simulink model "NUgus_IK"  (R2018a)
settings: Solver=VariableStepAuto  StartTime=0.0  StopTime=inf  RelTol=1e-3
values from neighbouring files (symbols this model uses):
  CM740_acc_bias = 4 * 9.80743    (= 39.22972)    [CM740_init.m]
  CM740_acc_gain = 512 / CM740_acc_centre    [CM740_init.m]
  CM740_gyro_bias = 1600 / 360 * 2 * pi    (= 27.9252680319)    [CM740_init.m]
  CM740_gyro_gain = 512 / CM740_gyro_centre    [CM740_init.m]
  head = [-0.05482228998067195, -0.00010888238321339966, 0.0011712900228573724, 0.41900000000000004]    [comtest.m]
  s = mean(abs(present_speed.data))    [RunServoTest.m]
  torso = [0.0050079703254699804, 0.008880921777563762, 0.1021503146237477, 2.5390000000000006]    [comtest.m]
undefined symbols (not defined in the file or in its folder): floor, X, Y, Z
libraries: sm_lib x211, fl_lib x128, nesl_utility x68
(part 8 of 8)

== system NUgus_IK/NUgus/left_foot/foot_fl_contact/calculate forces/x contact force ==
  PS Max1 : fl_lib/Physical Signals/Nonlinear Operators/PS Max
      settings: SourceProductName=Simscape  SourceProductBaseCode=SS
  PS Min1 : fl_lib/Physical Signals/Nonlinear Operators/PS Min
      settings: SourceProductName=Simscape  SourceProductBaseCode=SS
  PS Switch : fl_lib/Physical Signals/Nonlinear Operators/PS Switch  Threshold=0
      settings: SourceProductName=Simscape  SourceProductBaseCode=SS
  frictionless : PMIOPort  Side=Left
  force : PMIOPort  Port=2  Side=Right
  velocity : PMIOPort  Port=3  Side=Left
  z position : PMIOPort  Port=4  Side=Left
  upper_bound : PMIOPort  Port=5  Side=Left
  lower_bound : PMIOPort  Port=6  Side=Left
  connections:
  PS Max1/LConn2 -- lower_bound/RConn1
  PS Max1/LConn1 -- PS Min1/RConn1
  PS Switch/LConn3 -- PS Max1/RConn1
  PS Min1/LConn1 -- velocity/RConn1
  PS Switch/LConn2 -- z position/RConn1
  PS Switch/LConn1 -- frictionless/RConn1
  PS Switch/RConn1 -- force/RConn1
  upper_bound/RConn1 -- PS Min1/LConn2

== system NUgus_IK/NUgus/left_foot/foot_fl_contact/calculate forces/y contact force ==
  PS Max1 : fl_lib/Physical Signals/Nonlinear Operators/PS Max
      settings: SourceProductName=Simscape  SourceProductBaseCode=SS
  PS Min1 : fl_lib/Physical Signals/Nonlinear Operators/PS Min
      settings: SourceProductName=Simscape  SourceProductBaseCode=SS
  PS Switch : fl_lib/Physical Signals/Nonlinear Operators/PS Switch  Threshold=0
      settings: SourceProductName=Simscape  SourceProductBaseCode=SS
  frictionless : PMIOPort  Side=Left
  force : PMIOPort  Port=2  Side=Right
  velocity : PMIOPort  Port=3  Side=Left
  z position : PMIOPort  Port=4  Side=Left
  upper_bound : PMIOPort  Port=5  Side=Left
  lower_bound : PMIOPort  Port=6  Side=Left
  connections:
  PS Max1/LConn2 -- lower_bound/RConn1
  PS Max1/LConn1 -- PS Min1/RConn1
  PS Switch/LConn3 -- PS Max1/RConn1
  PS Min1/LConn1 -- velocity/RConn1
  PS Switch/LConn2 -- z position/RConn1
  PS Switch/LConn1 -- frictionless/RConn1
  PS Switch/RConn1 -- force/RConn1
  upper_bound/RConn1 -- PS Min1/LConn2

== system NUgus_IK/NUgus/left_foot/foot_fr_contact/calculate forces/x contact force ==
  PS Max1 : fl_lib/Physical Signals/Nonlinear Operators/PS Max
      settings: SourceProductName=Simscape  SourceProductBaseCode=SS
  PS Min1 : fl_lib/Physical Signals/Nonlinear Operators/PS Min
      settings: SourceProductName=Simscape  SourceProductBaseCode=SS
  PS Switch : fl_lib/Physical Signals/Nonlinear Operators/PS Switch  Threshold=0
      settings: SourceProductName=Simscape  SourceProductBaseCode=SS
  frictionless : PMIOPort  Side=Left
  force : PMIOPort  Port=2  Side=Right
  velocity : PMIOPort  Port=3  Side=Left
  z position : PMIOPort  Port=4  Side=Left
  upper_bound : PMIOPort  Port=5  Side=Left
  lower_bound : PMIOPort  Port=6  Side=Left
  connections:
  PS Max1/LConn2 -- lower_bound/RConn1
  PS Max1/LConn1 -- PS Min1/RConn1
  PS Switch/LConn3 -- PS Max1/RConn1
  PS Min1/LConn1 -- velocity/RConn1
  PS Switch/LConn2 -- z position/RConn1
  PS Switch/LConn1 -- frictionless/RConn1
  PS Switch/RConn1 -- force/RConn1
  upper_bound/RConn1 -- PS Min1/LConn2

== system NUgus_IK/NUgus/left_foot/foot_fr_contact/calculate forces/y contact force ==
  PS Max1 : fl_lib/Physical Signals/Nonlinear Operators/PS Max
      settings: SourceProductName=Simscape  SourceProductBaseCode=SS
  PS Min1 : fl_lib/Physical Signals/Nonlinear Operators/PS Min
      settings: SourceProductName=Simscape  SourceProductBaseCode=SS
  PS Switch : fl_lib/Physical Signals/Nonlinear Operators/PS Switch  Threshold=0
      settings: SourceProductName=Simscape  SourceProductBaseCode=SS
  frictionless : PMIOPort  Side=Left
  force : PMIOPort  Port=2  Side=Right
  velocity : PMIOPort  Port=3  Side=Left
  z position : PMIOPort  Port=4  Side=Left
  upper_bound : PMIOPort  Port=5  Side=Left
  lower_bound : PMIOPort  Port=6  Side=Left
  connections:
  PS Max1/LConn2 -- lower_bound/RConn1
  PS Max1/LConn1 -- PS Min1/RConn1
  PS Switch/LConn3 -- PS Max1/RConn1
  PS Min1/LConn1 -- velocity/RConn1
  PS Switch/LConn2 -- z position/RConn1
  PS Switch/LConn1 -- frictionless/RConn1
  PS Switch/RConn1 -- force/RConn1
  upper_bound/RConn1 -- PS Min1/LConn2

== system NUgus_IK/NUgus/right_foot/foot_bl_contact/calculate forces/x contact force ==
  PS Max1 : fl_lib/Physical Signals/Nonlinear Operators/PS Max
      settings: SourceProductName=Simscape  SourceProductBaseCode=SS
  PS Min1 : fl_lib/Physical Signals/Nonlinear Operators/PS Min
      settings: SourceProductName=Simscape  SourceProductBaseCode=SS
  PS Switch : fl_lib/Physical Signals/Nonlinear Operators/PS Switch  Threshold=0
      settings: SourceProductName=Simscape  SourceProductBaseCode=SS
  frictionless : PMIOPort  Side=Left
  force : PMIOPort  Port=2  Side=Right
  velocity : PMIOPort  Port=3  Side=Left
  z position : PMIOPort  Port=4  Side=Left
  upper_bound : PMIOPort  Port=5  Side=Left
  lower_bound : PMIOPort  Port=6  Side=Left
  connections:
  PS Max1/LConn2 -- lower_bound/RConn1
  PS Max1/LConn1 -- PS Min1/RConn1
  PS Switch/LConn3 -- PS Max1/RConn1
  PS Min1/LConn1 -- velocity/RConn1
  PS Switch/LConn2 -- z position/RConn1
  PS Switch/LConn1 -- frictionless/RConn1
  PS Switch/RConn1 -- force/RConn1
  upper_bound/RConn1 -- PS Min1/LConn2

== system NUgus_IK/NUgus/right_foot/foot_bl_contact/calculate forces/y contact force ==
  PS Max1 : fl_lib/Physical Signals/Nonlinear Operators/PS Max
      settings: SourceProductName=Simscape  SourceProductBaseCode=SS
  PS Min1 : fl_lib/Physical Signals/Nonlinear Operators/PS Min
      settings: SourceProductName=Simscape  SourceProductBaseCode=SS
  PS Switch : fl_lib/Physical Signals/Nonlinear Operators/PS Switch  Threshold=0
      settings: SourceProductName=Simscape  SourceProductBaseCode=SS
  frictionless : PMIOPort  Side=Left
  force : PMIOPort  Port=2  Side=Right
  velocity : PMIOPort  Port=3  Side=Left
  z position : PMIOPort  Port=4  Side=Left
  upper_bound : PMIOPort  Port=5  Side=Left
  lower_bound : PMIOPort  Port=6  Side=Left
  connections:
  PS Max1/LConn2 -- lower_bound/RConn1
  PS Max1/LConn1 -- PS Min1/RConn1
  PS Switch/LConn3 -- PS Max1/RConn1
  PS Min1/LConn1 -- velocity/RConn1
  PS Switch/LConn2 -- z position/RConn1
  PS Switch/LConn1 -- frictionless/RConn1
  PS Switch/RConn1 -- force/RConn1
  upper_bound/RConn1 -- PS Min1/LConn2

== system NUgus_IK/NUgus/right_foot/foot_br_contact/calculate forces/x contact force ==
  PS Max1 : fl_lib/Physical Signals/Nonlinear Operators/PS Max
      settings: SourceProductName=Simscape  SourceProductBaseCode=SS
  PS Min1 : fl_lib/Physical Signals/Nonlinear Operators/PS Min
      settings: SourceProductName=Simscape  SourceProductBaseCode=SS
  PS Switch : fl_lib/Physical Signals/Nonlinear Operators/PS Switch  Threshold=0
      settings: SourceProductName=Simscape  SourceProductBaseCode=SS
  frictionless : PMIOPort  Side=Left
  force : PMIOPort  Port=2  Side=Right
  velocity : PMIOPort  Port=3  Side=Left
  z position : PMIOPort  Port=4  Side=Left
  upper_bound : PMIOPort  Port=5  Side=Left
  lower_bound : PMIOPort  Port=6  Side=Left
  connections:
  PS Max1/LConn2 -- lower_bound/RConn1
  PS Max1/LConn1 -- PS Min1/RConn1
  PS Switch/LConn3 -- PS Max1/RConn1
  PS Min1/LConn1 -- velocity/RConn1
  PS Switch/LConn2 -- z position/RConn1
  PS Switch/LConn1 -- frictionless/RConn1
  PS Switch/RConn1 -- force/RConn1
  upper_bound/RConn1 -- PS Min1/LConn2

== system NUgus_IK/NUgus/right_foot/foot_br_contact/calculate forces/y contact force ==
  PS Max1 : fl_lib/Physical Signals/Nonlinear Operators/PS Max
      settings: SourceProductName=Simscape  SourceProductBaseCode=SS
  PS Min1 : fl_lib/Physical Signals/Nonlinear Operators/PS Min
      settings: SourceProductName=Simscape  SourceProductBaseCode=SS
  PS Switch : fl_lib/Physical Signals/Nonlinear Operators/PS Switch  Threshold=0
      settings: SourceProductName=Simscape  SourceProductBaseCode=SS
  frictionless : PMIOPort  Side=Left
  force : PMIOPort  Port=2  Side=Right
  velocity : PMIOPort  Port=3  Side=Left
  z position : PMIOPort  Port=4  Side=Left
  upper_bound : PMIOPort  Port=5  Side=Left
  lower_bound : PMIOPort  Port=6  Side=Left
  connections:
  PS Max1/LConn2 -- lower_bound/RConn1
  PS Max1/LConn1 -- PS Min1/RConn1
  PS Switch/LConn3 -- PS Max1/RConn1
  PS Min1/LConn1 -- velocity/RConn1
  PS Switch/LConn2 -- z position/RConn1
  PS Switch/LConn1 -- frictionless/RConn1
  PS Switch/RConn1 -- force/RConn1
  upper_bound/RConn1 -- PS Min1/LConn2

== system NUgus_IK/NUgus/right_foot/foot_fl_contact/calculate forces/x contact force ==
  PS Max1 : fl_lib/Physical Signals/Nonlinear Operators/PS Max
      settings: SourceProductName=Simscape  SourceProductBaseCode=SS
  PS Min1 : fl_lib/Physical Signals/Nonlinear Operators/PS Min
      settings: SourceProductName=Simscape  SourceProductBaseCode=SS
  PS Switch : fl_lib/Physical Signals/Nonlinear Operators/PS Switch  Threshold=0
      settings: SourceProductName=Simscape  SourceProductBaseCode=SS
  frictionless : PMIOPort  Side=Left
  force : PMIOPort  Port=2  Side=Right
  velocity : PMIOPort  Port=3  Side=Left
  z position : PMIOPort  Port=4  Side=Left
  upper_bound : PMIOPort  Port=5  Side=Left
  lower_bound : PMIOPort  Port=6  Side=Left
  connections:
  PS Max1/LConn2 -- lower_bound/RConn1
  PS Max1/LConn1 -- PS Min1/RConn1
  PS Switch/LConn3 -- PS Max1/RConn1
  PS Min1/LConn1 -- velocity/RConn1
  PS Switch/LConn2 -- z position/RConn1
  PS Switch/LConn1 -- frictionless/RConn1
  PS Switch/RConn1 -- force/RConn1
  upper_bound/RConn1 -- PS Min1/LConn2

== system NUgus_IK/NUgus/right_foot/foot_fl_contact/calculate forces/y contact force ==
  PS Max1 : fl_lib/Physical Signals/Nonlinear Operators/PS Max
      settings: SourceProductName=Simscape  SourceProductBaseCode=SS
  PS Min1 : fl_lib/Physical Signals/Nonlinear Operators/PS Min
      settings: SourceProductName=Simscape  SourceProductBaseCode=SS
  PS Switch : fl_lib/Physical Signals/Nonlinear Operators/PS Switch  Threshold=0
      settings: SourceProductName=Simscape  SourceProductBaseCode=SS
  frictionless : PMIOPort  Side=Left
  force : PMIOPort  Port=2  Side=Right
  velocity : PMIOPort  Port=3  Side=Left
  z position : PMIOPort  Port=4  Side=Left
  upper_bound : PMIOPort  Port=5  Side=Left
  lower_bound : PMIOPort  Port=6  Side=Left
  connections:
  PS Max1/LConn2 -- lower_bound/RConn1
  PS Max1/LConn1 -- PS Min1/RConn1
  PS Switch/LConn3 -- PS Max1/RConn1
  PS Min1/LConn1 -- velocity/RConn1
  PS Switch/LConn2 -- z position/RConn1
  PS Switch/LConn1 -- frictionless/RConn1
  PS Switch/RConn1 -- force/RConn1
  upper_bound/RConn1 -- PS Min1/LConn2

== system NUgus_IK/NUgus/right_foot/foot_fr_contact/calculate forces/x contact force ==
  PS Max1 : fl_lib/Physical Signals/Nonlinear Operators/PS Max
      settings: SourceProductName=Simscape  SourceProductBaseCode=SS
  PS Min1 : fl_lib/Physical Signals/Nonlinear Operators/PS Min
      settings: SourceProductName=Simscape  SourceProductBaseCode=SS
  PS Switch : fl_lib/Physical Signals/Nonlinear Operators/PS Switch  Threshold=0
      settings: SourceProductName=Simscape  SourceProductBaseCode=SS
  frictionless : PMIOPort  Side=Left
  force : PMIOPort  Port=2  Side=Right
  velocity : PMIOPort  Port=3  Side=Left
  z position : PMIOPort  Port=4  Side=Left
  upper_bound : PMIOPort  Port=5  Side=Left
  lower_bound : PMIOPort  Port=6  Side=Left
  connections:
  PS Max1/LConn2 -- lower_bound/RConn1
  PS Max1/LConn1 -- PS Min1/RConn1
  PS Switch/LConn3 -- PS Max1/RConn1
  PS Min1/LConn1 -- velocity/RConn1
  PS Switch/LConn2 -- z position/RConn1
  PS Switch/LConn1 -- frictionless/RConn1
  PS Switch/RConn1 -- force/RConn1
  upper_bound/RConn1 -- PS Min1/LConn2

== system NUgus_IK/NUgus/right_foot/foot_fr_contact/calculate forces/y contact force ==
  PS Max1 : fl_lib/Physical Signals/Nonlinear Operators/PS Max
      settings: SourceProductName=Simscape  SourceProductBaseCode=SS
  PS Min1 : fl_lib/Physical Signals/Nonlinear Operators/PS Min
      settings: SourceProductName=Simscape  SourceProductBaseCode=SS
  PS Switch : fl_lib/Physical Signals/Nonlinear Operators/PS Switch  Threshold=0
      settings: SourceProductName=Simscape  SourceProductBaseCode=SS
  frictionless : PMIOPort  Side=Left
  force : PMIOPort  Port=2  Side=Right
  velocity : PMIOPort  Port=3  Side=Left
  z position : PMIOPort  Port=4  Side=Left
  upper_bound : PMIOPort  Port=5  Side=Left
  lower_bound : PMIOPort  Port=6  Side=Left
  connections:
  PS Max1/LConn2 -- lower_bound/RConn1
  PS Max1/LConn1 -- PS Min1/RConn1
  PS Switch/LConn3 -- PS Max1/RConn1
  PS Min1/LConn1 -- velocity/RConn1
  PS Switch/LConn2 -- z position/RConn1
  PS Switch/LConn1 -- frictionless/RConn1
  PS Switch/RConn1 -- force/RConn1
  upper_bound/RConn1 -- PS Min1/LConn2

== matlab function NUgus_IK/Forward Kinematics/Simulink Function/FK Function ==
  data: HtRSp output; p input; HtLSp output; HtRSr output; HtLSr output; HtRE output; HtLE output; HtRHy output; HtLHy output; HtRHr output; HtLHr output; HtRHp output; HtLHp output; HtRK output; HtLK output; HtRAp output; HtLAp output; HtRAr output; HtLAr output; HtHy output; HtHp output
function [HtRSp, HtLSp, HtRSr, HtLSr, HtRE, HtLE, HtRHy, HtLHy, HtRHr, HtLHr, HtRHp, HtLHp, HtRK, HtLK, HtRAp, HtLAp, HtRAr, HtLAr, HtHy, HtHp] = FK(p)
    model = NUgusKinematics();

    kinematics = Kinematics(model);
    
    % Get FK for arms
    [RSp, RSr, RE] = kinematics.armFK(p, false);
    [LSp, LSr, LE] = kinematics.armFK(p, true);
    % Get FK for legs
    [RHy, RHr, RHp, RK, RAp, RAr] = kinematics.legFK(p, false);
    [LHy, LHr, LHp, LK, LAp, LAr] = kinematics.legFK(p, true);
    % Get FK for Head
    [Hy, Hp] = kinematics.headFK(p);
    
    % Return FK in servo order
    HtRSp = RSp.tf;
    HtLSp = LSp.tf;
    HtRSr = RSr.tf;
    HtLSr = LSr.tf;
    HtRE = RE.tf;
    HtLE = LE.tf;
    HtRHy = RHy.tf;
    HtLHy = LHy.tf;
    HtRHr = RHr.tf;
    HtLHr = LHr.tf;
    HtRHp = RHp.tf;
    HtLHp = LHp.tf;
    HtRK = RK.tf;
    HtLK = LK.tf;
    HtRAp = RAp.tf;
    HtLAp = LAp.tf;
    HtRAr = RAr.tf;
    HtLAr = LAr.tf;
    HtHy = Hy.tf;
    HtHp = Hp.tf;
end

== matlab function NUgus_IK/Inverse Kinematics/Simulink Function/IK Function ==
  data: thetaTRSp output; rTRh input; rTLh input; HTRl input; HTLl input; rCP input; thetaTLSp output; thetaTRSr output; thetaTLSr output; thetaTRE output; thetaTLE output; thetaTRHy output; thetaTLHy output; thetaTRHr output; thetaTLHr output; thetaTRHp output; thetaTLHp output; thetaTRK output; thetaTLK output; thetaTRAp output; thetaTLAp output; thetaTRAr output; thetaTLAr output; thetaTNy output; thetaTNp output
function [thetaTRSp, thetaTLSp, thetaTRSr, thetaTLSr, thetaTRE, thetaTLE, thetaTRHy, thetaTLHy, thetaTRHr, thetaTLHr, thetaTRHp, thetaTLHp, thetaTRK, thetaTLK, thetaTRAp, thetaTLAp, thetaTRAr, thetaTLAr, thetaTNy, thetaTNp] = IK(rTRh, rTLh, HTRl, HTLl, rCP)
    model = NUgusKinematics();
    
    kinematics = Kinematics(model);

    % Head IK
    [thetaTNy, thetaTNp] = kinematics.headIK(rCP);
    % Arm IK
    [thetaTRSp, thetaTRSr, thetaTRE] = kinematics.armIK(rTRh, false);
    [thetaTLSp, thetaTLSr, thetaTLE] = kinematics.armIK(rTLh, true);

    % Leg IK
    [thetaTRHy, thetaTRHr, thetaTRHp, thetaTRK, thetaTRAp, thetaTRAr] = kinematics.legIK(HTRl, false);
    [thetaTLHy, thetaTLHr, thetaTLHp, thetaTLK, thetaTLAp, thetaTLAr] = kinematics.legIK(HTLl, true);

    %p = kinematics.getIK(rTRh, rTLh, HTRl, HTLl, rCP);
end
